simulink model "velo_id_gain_sl"  (R2023b)
settings: Solver=FixedStepDiscrete  StartTime=0.0  StopTime=10.0  FixedStep=1/50  RelTol=1e-3  EnableMultiTasking=on
values from neighbouring files (symbols this model uses):
  ts = 1/50    (= 0.02)    [velo_id_gain.m]    (also in velo_id_gain_cp.m; velo_id_tc.m; velo_pi_mbd.m)
  u_ini = 1.5    [velo_id_gain.m]    (also in velo_id_gain_cp.m; velo_id_tc.m = 3)
  u_ref = u_ref_list(i)    [velo_id_gain.m]
libraries: arduinolib x2
settings Model: ExtModeTrigDuration=2  Creator=MunoLike  LastModifiedBy=MunoLike
settings DataIOCC: SaveFormat=Array  SaveOutput=off  ReturnWorkspaceOutputs=off
settings OptimizationCC: EnhancedBackFolding=on  PassReuseOutputArgsAs=Individual arguments  ZeroExternalMemoryAtStartup=off  ZeroInternalMemoryAtStartup=off  MaxStackSize=64  OptimizeBlockOrder=speed  DifferentSizesBufferReuse=on  OptimizationCustomize=off  EfficientTunableParamExpr=on
settings DebuggingCC: ParameterTunabilityLossMsg=error
settings HardwareCC: ProdBitPerInt=16  ProdBitPerPointer=16  ProdBitPerSizeT=16  ProdBitPerPtrDiffT=16  ProdLargestAtomicFloat=None  ProdWordSize=8  ProdHWDeviceType=Atmel->AVR  UseEmbeddedCoderFeatures=off  UseSimulinkCoderFeatures=off
settings SFSimCC: MATLABDynamicMemAlloc=off
settings RTWCC: Description=Embedded Coder  SystemTargetFile=ert.tlc  HardwareBoard=Arduino Uno  TemplateMakefile=ert_default_tmf  Toolchain=Arduino AVR  BuildConfiguration=Faster Runs
settings CodeAppCC: ForceParamTrailComments=on  IgnoreCustomStorageClasses=off  OperatorAnnotations=on  SimulinkDataObjDesc=on  SFDataObjDesc=on  InsertBlockDesc=on
settings ERTTargetCC: SupportContinuousTime=on  SupportNonInlinedSFcns=on  SupportVariableSizeSignals=on  ExtModeTransport=3  ExtModeStaticAlloc=on  ExtModeAutomaticAllocSize=off  ExtModeStaticAllocSize=250  ExtModeMexFile=ext_xcp  ExtModeIntrfLevel=Level2 - Open

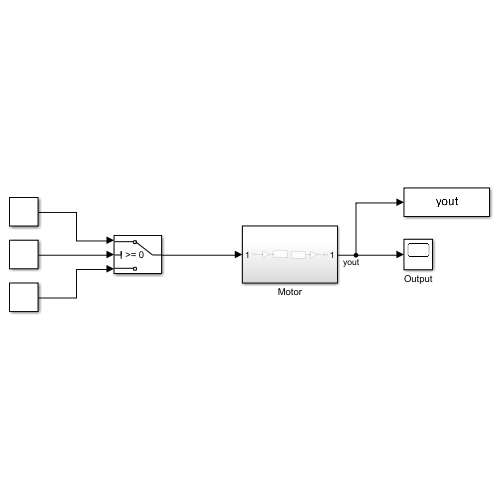
[thumbnail: Simulink's stored preview of the top-level diagram]
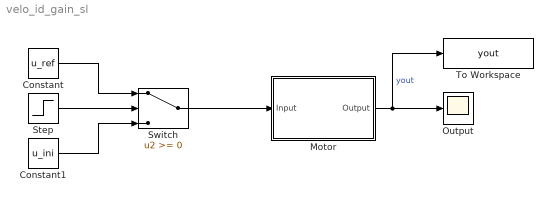
== system velo_id_gain_sl ==
  Constant : Constant  Value=u_ref
  Constant1 : Constant  Value=u_ini
  Motor : Subsystem
  Output : Scope
  Step : Step  SampleTime=0
  Switch : Switch  SaturateOnIntegerOverflow=off  InputSameDT=off
  To Workspace : ToWorkspace  VariableName=yout  SaveFormat=Structure With Time  SampleTime=-1
  wires:
  Constant/1 -> Switch/1
  Step/1 -> Switch/2
  Constant1/1 -> Switch/3
  Switch/1 -> Motor/1(Input)
  Motor/1(Output) -> To Workspace/1, Output/1  "yout"

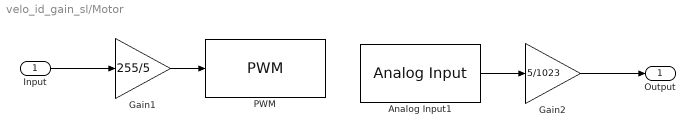
== system velo_id_gain_sl/Motor ==
  Input : Inport
  Analog Input1 : arduinolib/Analog Input  pinNumber=0  ReadResultsOnly=off  ConversionTriggerSource=Software  ExternalTriggerType=uint32( 0 )  OutputDataType=uint16  EnableConversionCompleteNotify=off  EnableOuputStatus=off  SampleTime=ts  blockPlatform=arduino
  Gain1 : Gain  Gain=255/5  OutDataTypeStr=double
  Gain2 : Gain  Gain=5/1023  OutDataTypeStr=double
  PWM : arduinolib/PWM  pinNumber=3  frequencyType=Default  desiredFrequency=490.2  achievableFrequency=490.2
  Output : Outport
  wires:
  Input/1 -> Gain1/1
  Analog Input1/1 -> Gain2/1
  Gain1/1 -> PWM/1
  Gain2/1 -> Output/1
